simulink model "P1_Ex3"  (R2021a)
settings: Solver=FixedStepAuto  StartTime=0.0  StopTime=Total_time  RelTol=1e-3
PreLoadFcn:
  | PreLoad_P1_Ex3
StopFcn:
  | post_P1_Ex3
values from neighbouring files (symbols this model uses):
  Kp = 2    [PreLoad_P1_Ex3.m]
  Tg = 0.005    [PreLoad_P1_Ex3.m]
  Ts = 0.01    [PreLoad_P1_Ex3.m]
libraries: arduinolib x5, simulink x1
settings Model: SimulationMode=external  ExtModeTrigDuration=2  Creator=Eneko Lerma  LastModifiedBy=Control Automatic
settings SolverCC: AlgebraicLoopSolver=TrustRegion
settings DataIOCC: ReturnWorkspaceOutputs=off
settings OptimizationCC: EnhancedBackFolding=on  PassReuseOutputArgsAs=Individual arguments  MaxStackSize=64  OptimizeBlockOrder=speed  DifferentSizesBufferReuse=on  OptimizationCustomize=off  EfficientTunableParamExpr=on
settings DebuggingCC: ParameterPrecisionLossMsg=none  ParameterTunabilityLossMsg=error  SFMachineParentedDataDiag=warning  ArithmeticOperatorsInVariantConditions=warning
settings HardwareCC: ProdBitPerPointer=32  ProdBitPerSizeT=32  ProdBitPerPtrDiffT=32  ProdLargestAtomicInteger=Long  ProdLargestAtomicFloat=Double  ProdWordSize=32  ProdHWDeviceType=ARM Compatible->ARM Cortex
settings SFSimCC: SimUseLocalCustomCode=off  MATLABDynamicMemAlloc=off  CustomCodeUndefinedFunction=UseInterfaceOnly
settings RTWCC: SystemTargetFile=ert.tlc  HardwareBoard=Arduino Due  TemplateMakefile=ert_default_tmf  GenerateReport=on  RTWUseLocalCustomCode=off  Toolchain=Arduino ARM  BuildConfiguration=Faster Runs  IncludeHyperlinkInReport=on  LaunchReport=on  GenerateTraceInfo=on  GenerateTraceReport=on  GenerateTraceReportSl=on  GenerateTraceReportSf=on  GenerateTraceReportEml=on
settings RTWCC: CustomTerminator=|
  | writeDigitalPin((uint8_T)3, 0);
  | writeDigitalPin((uint8_T)5, 0);
settings CodeAppCC: ForceParamTrailComments=on  IgnoreCustomStorageClasses=off  OperatorAnnotations=on  SimulinkDataObjDesc=on  SFDataObjDesc=on  InsertBlockDesc=on
settings ERTTargetCC: SupportContinuousTime=on  SupportVariableSizeSignals=on

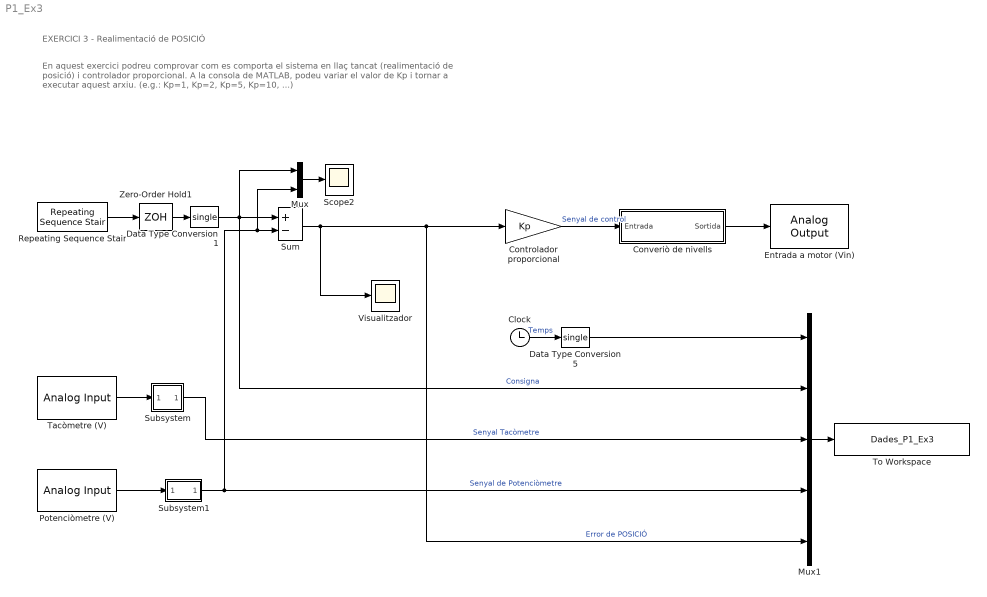
== system P1_Ex3 ==
  note: EXERCICI 3 - Realimentació de POSICIÓ
  note: En aquest exercici podreu comprovar com es comporta el sistema en llaç tancat (realimentació de posició)
      | i controlador proporcional. A la consola de MATLAB, podeu variar el valor de Kp i tornar a executar aquest arxiu.
      | (e.g.: Kp=1, Kp=2, Kp=5, Kp=10, ...)
  Clock : Clock
  Controlador proporcional : Gain  Gain=Kp
  Converiò de nivells : Subsystem
  Data Type Conversion1 : DataTypeConversion  OutDataTypeStr=single
  Data Type Conversion5 : DataTypeConversion  OutDataTypeStr=single
  Entrada a motor (Vin) : arduinolib/Analog Output  DACpin=DAC1  blockPlatform=arduino
      settings: SourceProductBaseCode=ARDUINO
  Mux : Mux  Inputs=2
  Mux1 : Mux  Inputs=5
  Potenciòmetre (V) : arduinolib/Analog Input  pinNumber=1  ReadResultsOnly=off  ConversionTriggerSource=Software  ExternalTriggerType=uint32(0)  OutputDataType=uint16  EnableConversionCompleteNotify=off  EnableOuputStatus=off  SampleTime=Tg  blockPlatform=arduino
  Repeating Sequence Stair : simulink/Sources/Repeating Sequence Stair  OutValues=input_vector  tsamp=t  OutMin=[]  OutMax=[]  OutDataTypeStr=float('double')  OutputDataTypeScalingMode=Specify via dialog  OutDataType=float('double')  ConRadixGroup=Best Precision: Vector-wise  OutScaling=2^-12
  Scope2 : Scope
  Subsystem : Subsystem
  Subsystem1 : Subsystem
  Sum : Sum  Inputs=+-
  Tacòmetre (V) : arduinolib/Analog Input  pinNumber=0  ReadResultsOnly=off  ConversionTriggerSource=Software  ExternalTriggerType=uint32(0)  OutputDataType=uint16  EnableConversionCompleteNotify=off  EnableOuputStatus=off  SampleTime=Tg  blockPlatform=arduino
  To Workspace : ToWorkspace  VariableName=Dades_P1_Ex3  SampleTime=-1
  Visualitzador : Scope
  Zero-Order Hold1 : ZeroOrderHold  SampleTime=Ts
  wires:
  Mux/1 -> Scope2/1
  Controlador proporcional/1 -> Converiò de nivells/1(Entrada)  "Senyal de control"
  Converiò de nivells/1(Sortida) -> Entrada a motor (Vin)/1
  Zero-Order Hold1/1 -> Data Type Conversion1/1
  Sum/1 -> Visualitzador/1, Mux1/5, Controlador proporcional/1  "Error de POSICIÓ"
  Data Type Conversion1/1 -> Mux1/2, Sum/1, Mux/1  "Consigna"
  Mux1/1 -> To Workspace/1
  Clock/1 -> Data Type Conversion5/1  "Temps"
  Data Type Conversion5/1 -> Mux1/1
  Repeating Sequence Stair/1 -> Zero-Order Hold1/1
  Tacòmetre (V)/1 -> Subsystem/1("    ")
  Subsystem/1("       ") -> Mux1/3  "Senyal Tacòmetre"
  Subsystem1/1("     ") -> Mux/2, Sum/2, Mux1/4  "Senyal de Potenciòmetre"
  Potenciòmetre (V)/1 -> Subsystem1/1("    ")

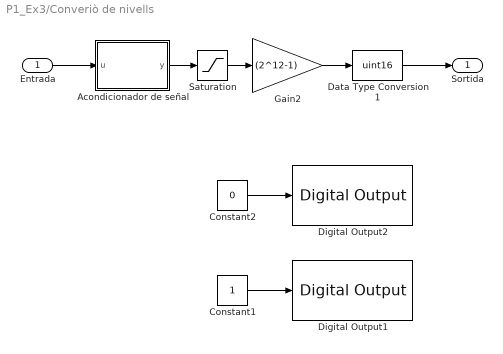
== system P1_Ex3/Converiò de nivells ==
  Entrada : Inport  OutDataTypeStr=single
  Acondicionador de señal : MATLAB Function  TreatAsAtomicUnit=on
  Constant1 : Constant
  Constant2 : Constant  Value=0
  Data Type Conversion1 : DataTypeConversion  OutDataTypeStr=uint16
  Digital Output1 : arduinolib/Digital Output  pinNumber=5  Direction=output  blockPlatform=arduino
  Digital Output2 : arduinolib/Digital Output  pinNumber=3  Direction=output  blockPlatform=arduino
  Gain2 : Gain  Gain=(2^12-1)  OutDataTypeStr=single
  Saturation : Saturate  UpperLimit=1  LowerLimit=0  OutDataTypeStr=single
  Sortida : Outport  OutDataTypeStr=uint16  VectorParamsAs1DForOutWhenUnconnected=off
  wires:
  Gain2/1 -> Data Type Conversion1/1
  Entrada/1 -> Acondicionador de señal/1(u)
  Acondicionador de señal/1(y) -> Saturation/1
  Data Type Conversion1/1 -> Sortida/1
  Saturation/1 -> Gain2/1
  Constant2/1 -> Digital Output2/1
  Constant1/1 -> Digital Output1/1

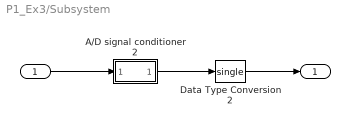
== system P1_Ex3/Subsystem ==
  "    " : Inport
  A/D signal conditioner2 : Subsystem
  Data Type Conversion2 : DataTypeConversion  OutDataTypeStr=single
  "       " : Outport  VectorParamsAs1DForOutWhenUnconnected=off
  wires:
  A/D signal conditioner2/1(" ") -> Data Type Conversion2/1
  Data Type Conversion2/1 -> "       "/1
  "    "/1 -> A/D signal conditioner2/1(" ")

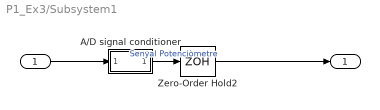
== system P1_Ex3/Subsystem1 ==
  "    " : Inport
  A/D signal conditioner : Subsystem
  Zero-Order Hold2 : ZeroOrderHold  SampleTime=Ts
  "     " : Outport  VectorParamsAs1DForOutWhenUnconnected=off
  wires:
  A/D signal conditioner/1(" ") -> Zero-Order Hold2/1  "Senyal Potenciòmetre"
  "    "/1 -> A/D signal conditioner/1(" ")
  Zero-Order Hold2/1 -> "     "/1

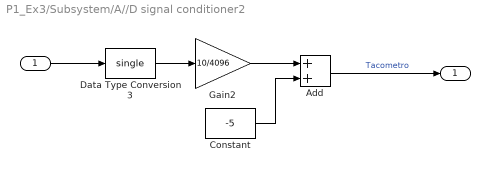
== system P1_Ex3/Subsystem/A//D signal conditioner2 ==
  " " : Inport
  Add : Sum  AccumDataTypeStr=single
  Constant : Constant  Value=-5  OutDataTypeStr=single
  Data Type Conversion3 : DataTypeConversion  OutDataTypeStr=single
  Gain2 : Gain  Gain=10/4096  OutDataTypeStr=single
  " " : Outport  VectorParamsAs1DForOutWhenUnconnected=off
  wires:
  " "/1 -> Data Type Conversion3/1
  Add/1 -> " "/1  "Tacometro"
  Gain2/1 -> Add/1
  Constant/1 -> Add/2
  Data Type Conversion3/1 -> Gain2/1

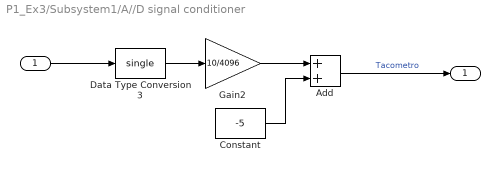
== system P1_Ex3/Subsystem1/A//D signal conditioner ==
  " " : Inport
  Add : Sum  AccumDataTypeStr=single
  Constant : Constant  Value=-5  OutDataTypeStr=single
  Data Type Conversion3 : DataTypeConversion  OutDataTypeStr=single
  Gain2 : Gain  Gain=10/4096  OutDataTypeStr=single
  " " : Outport  VectorParamsAs1DForOutWhenUnconnected=off
  wires:
  Data Type Conversion3/1 -> Gain2/1
  Constant/1 -> Add/2
  Gain2/1 -> Add/1
  Add/1 -> " "/1  "Tacometro"
  " "/1 -> Data Type Conversion3/1

== matlab function P1_Ex3/Converiò de nivells/Acondicionador de señal ==
  data: u input; y output
function y = fcn(u)
y =0.0968*u+0.5058;
